simulink model "exercise_2_2"  (R2024b)
settings: Solver=VariableStepAuto  StartTime=0.0  StopTime=30  RelTol=1e-3
InitFcn:
  | disp('Loading EMG data...');
  | data = load('ES2_emg.mat');
  | 
  | signals = data.ES2_emg.signals; %30001x4
  | 
  | % Create time vector
  | Ts = 0.001;
  | 
  | num_samples = size(signals, 1);
  | 
  | time_vector = (0:num_samples-1)' * Ts;
  | 
  | raw_signals = [time_vector, signals];     % [Time, Data] 30001x5
  | 
  | disp('Data loaded and time vector created.');
  | 
  | 
  | %% FILTER DESIGN
  | 
  | Fs = 1/Ts;     % 1000 Hz
  | 
  | disp('Designing filters ...');
  | 
  | % NOTCH FILTER (50 Hz)
  | f0 = 50;
  | Q = 40;        % quality factor: higher means narrower notch
  | BW = f0 / Q;
  | d_notch = designfilt('bandstopiir', ...
  |     'FilterOrder', 2, ...
  |     'HalfPowerFrequency1', f0 - BW/2, ...
  |     'HalfPowerFrequency2', f0 + BW/2, ...
  |     'DesignMethod', 'butter', ...
  |     'SampleRate', Fs);
  | [b_notch, a_notch] = tf(d_notch);
  | 
  | % BANDPASS FILTER (30–450 Hz)
  | d_band = designfilt('bandpassiir', ...
  |     'FilterOrder', 4, ...
  |     'HalfPowerFrequency1', 30, ...
  |     'HalfPowerFrequency2', 450, ...
  |     'DesignMethod', 'butter', ...
  |     'SampleRate', Fs);
  | [b_band, a_band] = tf(d_band);
  | 
  | % LOWPASS FILTER (0.8 Hz)
  | d_low = designfilt('lowpassiir', ...
  |     'FilterOrder', 4, ...
  |     'HalfPowerFrequency', 0.8, ...
  |     'DesignMethod', 'butter', ...
  |     'SampleRate', Fs);
  | [b_low, a_low] = tf(d_low);
  | 
  | % LOWPASS AFTER DIVISION
  | f_cutoff = 0.5;
  | d_lowpass = designfilt('lowpassiir', ...
  |     'FilterOrder', 2, ...
  |     'HalfPowerFrequency', f_cutoff, ...
  |     'DesignMethod', 'butter', ...
  |     'SampleRate', Fs);
  | [b_low2, a_low2] = tf(d_lowpass);
  | 
  | disp('Filter coefficients generated');
undefined symbols (not defined in the file or in its folder): a_band, a_low, a_low2, a_notch, b_band, b_low, b_low2, b_notch, dspblkCoreblockFVToolHelper, gcbh
libraries: vrlib x1
settings Model: Creator=Lenovo  LastModifiedBy=philg
settings RTWCC: GPUComputeCapability=3.5

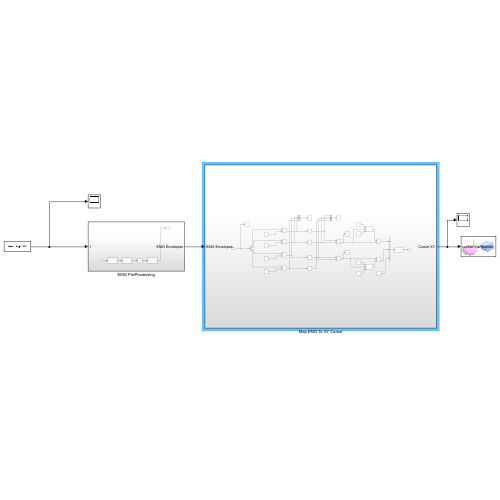
[thumbnail: Simulink's stored preview of the top-level diagram]
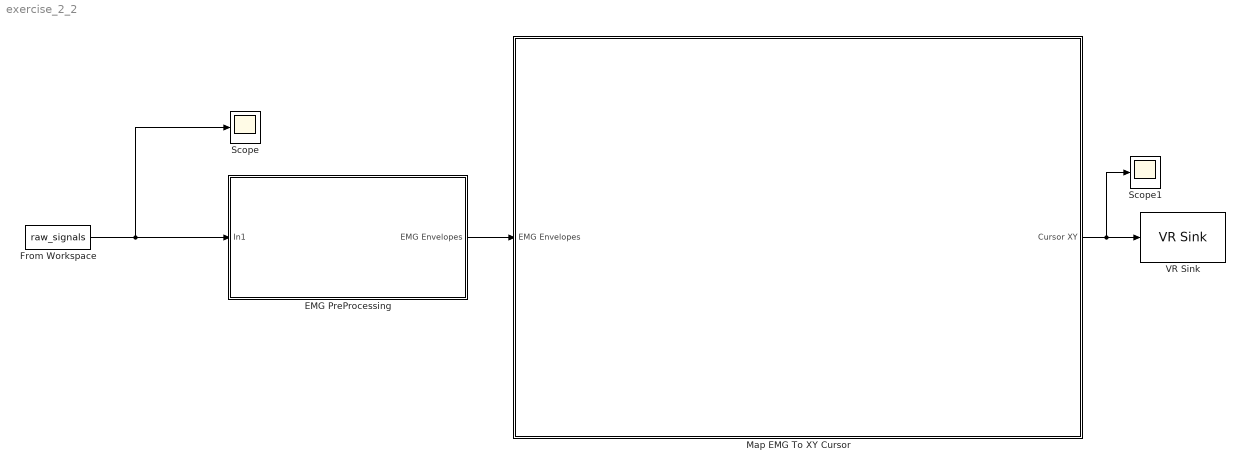
== system exercise_2_2 ==
  EMG PreProcessing : Subsystem
  From Workspace : FromWorkspace  VariableName=raw_signals  SampleTime=0.001  Interpolate=off  ZeroCross=off  OutputAfterFinalValue=Holding final value
  Map EMG To XY Cursor : Subsystem
  Scope : Scope
  Scope1 : Scope
  VR Sink : vrlib/VR Sink  InstantiateOnLoad=on  SampleTime=0.1  ViewEnable=on  RemoteChange=off  RemoteView=off  FieldsWritten=cursor.translation.3.1.1.double  WorldFileName=8_palline_color.wrl  AutoView=off  VideoDimensions=[]  AllowVariableSize=off
  wires:
  From Workspace/1 -> EMG PreProcessing/1(In1), Scope/1
  EMG PreProcessing/1(EMG Envelopes) -> Map EMG To XY Cursor/1(EMG Envelopes)
  Map EMG To XY Cursor/1(Cursor XY) -> VR Sink/1, Scope1/1

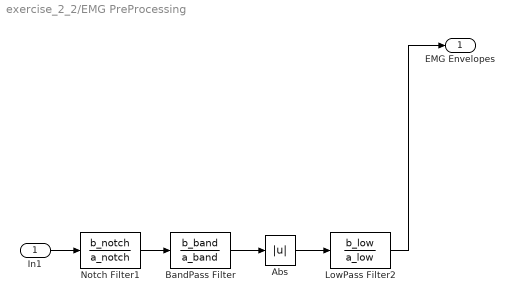
== system exercise_2_2/EMG PreProcessing ==
  In1 : Inport
  Abs : Abs  SaturateOnIntegerOverflow=off
  BandPass Filter : DiscreteFilter  LoadFcn=dspblkCoreblockFVToolHelper(gcbh,'load');  Numerator=b_band  Denominator=a_band
      settings: CopyFcn=dspblkCoreblockFVToolHelper(gcbh,'copy');  DeleteFcn=dspblkCoreblockFVToolHelper(gcbh,'close');  ModelCloseFcn=dspblkCoreblockFVToolHelper(gcbh,'close');  PreSaveFcn=dspblkCoreblockFVToolHelper(gcbh,'presave');  PostSaveFcn=dspblkCoreblockFVToolHelper(gcbh,'postsave');  CloseFcn=dspblkCoreblockFVToolHelper(gcbh,'close');
  LowPass Filter2 : DiscreteFilter  Numerator=b_low  Denominator=a_low
  Notch Filter1 : DiscreteFilter  LoadFcn=dspblkCoreblockFVToolHelper(gcbh,'load');  Numerator=b_notch  Denominator=a_notch
      settings: CopyFcn=dspblkCoreblockFVToolHelper(gcbh,'copy');  DeleteFcn=dspblkCoreblockFVToolHelper(gcbh,'close');  ModelCloseFcn=dspblkCoreblockFVToolHelper(gcbh,'close');  PreSaveFcn=dspblkCoreblockFVToolHelper(gcbh,'presave');  PostSaveFcn=dspblkCoreblockFVToolHelper(gcbh,'postsave');  CloseFcn=dspblkCoreblockFVToolHelper(gcbh,'close');
  EMG Envelopes : Outport
  wires:
  Abs/1 -> LowPass Filter2/1
  In1/1 -> Notch Filter1/1
  Notch Filter1/1 -> BandPass Filter/1
  BandPass Filter/1 -> Abs/1
  LowPass Filter2/1 -> EMG Envelopes/1

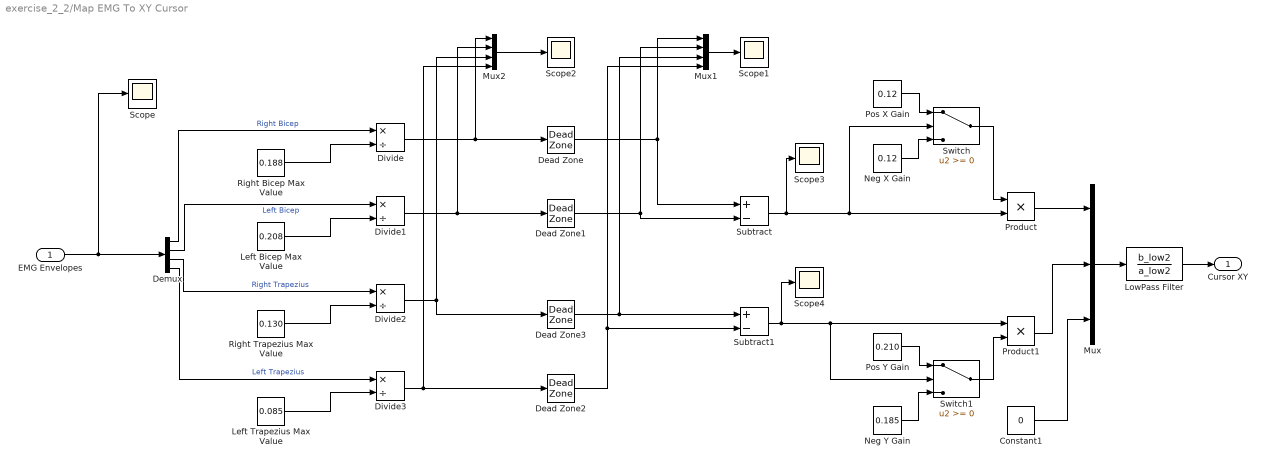
== system exercise_2_2/Map EMG To XY Cursor ==
  EMG Envelopes : Inport
  Constant1 : Constant  Value=0
  Dead Zone : DeadZone  LowerValue=0  UpperValue=0.1
  Dead Zone1 : DeadZone  LowerValue=0  UpperValue=0.1
  Dead Zone2 : DeadZone  LowerValue=0  UpperValue=0.4
  Dead Zone3 : DeadZone  LowerValue=0  UpperValue=0.3
  Demux : Demux
  Divide{,1..3} (4 alike) : Product  Inputs=*/
  Left Bicep Max Value : Constant  Value=0.208
  Left Trapezius Max Value : Constant  Value=0.085
  LowPass Filter : DiscreteFilter  LoadFcn=dspblkCoreblockFVToolHelper(gcbh,'load');  Numerator=b_low2  Denominator=a_low2
      settings: CopyFcn=dspblkCoreblockFVToolHelper(gcbh,'copy');  DeleteFcn=dspblkCoreblockFVToolHelper(gcbh,'close');  ModelCloseFcn=dspblkCoreblockFVToolHelper(gcbh,'close');  PreSaveFcn=dspblkCoreblockFVToolHelper(gcbh,'presave');  PostSaveFcn=dspblkCoreblockFVToolHelper(gcbh,'postsave');  CloseFcn=dspblkCoreblockFVToolHelper(gcbh,'close');
  Mux : Mux  Inputs=3
  Mux1 : Mux
  Mux2 : Mux
  Neg X Gain : Constant  Value=0.12
  Neg Y Gain : Constant  Value=0.185
  Pos X Gain : Constant  Value=0.12
  Pos Y Gain : Constant  Value=0.210
  Product : Product
  Product1 : Product
  Right Bicep Max Value : Constant  Value=0.188
  Right Trapezius Max Value : Constant  Value=0.130
  Scope{,1..4} (5 alike) : Scope
  Subtract : Sum  Inputs=+-
  Subtract1 : Sum  Inputs=+-
  Switch : Switch  SaturateOnIntegerOverflow=off  InputSameDT=off
  Switch1 : Switch  SaturateOnIntegerOverflow=off  InputSameDT=off
  Cursor XY : Outport
  wires:
  Constant1/1 -> Mux/3
  Demux/3 -> Divide2/1  "Right Trapezius"
  Demux/2 -> Divide1/1  "Left Bicep"
  Demux/4 -> Divide3/1  "Left Trapezius"
  Demux/1 -> Divide/1  "Right Bicep"
  EMG Envelopes/1 -> Scope/1, Demux/1
  Mux/1 -> LowPass Filter/1
  Mux1/1 -> Scope1/1
  Right Bicep Max Value/1 -> Divide/2
  Left Bicep Max Value/1 -> Divide1/2
  Right Trapezius Max Value/1 -> Divide2/2
  Left Trapezius Max Value/1 -> Divide3/2
  LowPass Filter/1 -> Cursor XY/1
  Divide/1 -> Mux2/1, Dead Zone/1
  Divide1/1 -> Mux2/2, Dead Zone1/1
  Divide2/1 -> Mux2/3, Dead Zone3/1
  Divide3/1 -> Mux2/4, Dead Zone2/1
  Mux2/1 -> Scope2/1
  Dead Zone/1 -> Mux1/1, Subtract/1
  Dead Zone1/1 -> Mux1/2, Subtract/2
  Subtract/1 -> Scope3/1, Switch/2, Product/2
  Subtract1/1 -> Switch1/2, Product1/1, Scope4/1
  Dead Zone3/1 -> Mux1/3, Subtract1/1
  Dead Zone2/1 -> Mux1/4, Subtract1/2
  Product/1 -> Mux/1
  Switch/1 -> Product/1
  Switch1/1 -> Product1/2
  Product1/1 -> Mux/2
  Neg X Gain/1 -> Switch/3
  Pos X Gain/1 -> Switch/1
  Pos Y Gain/1 -> Switch1/1
  Neg Y Gain/1 -> Switch1/3
